simulink subsystem "SubSysWrappedState_Simplified7DOF"  (R2019b)
settings: Solver=VariableStepAuto  StartTime=0.0  StopTime=10.0  RelTol=1e-3
undefined symbols (not defined in the file): psi, psidot, X, xdot, Y, ydot
settings Model: Creator=yeyuan  LastModifiedBy=yeyuan

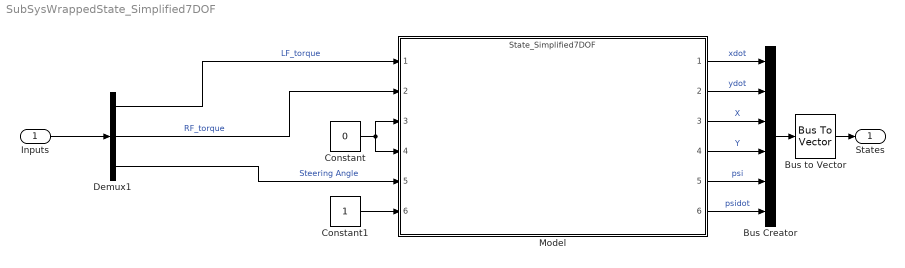
== system SubSysWrappedState_Simplified7DOF ==
  Inputs : Inport
  Bus Creator : BusCreator  Inputs=xdot,ydot,X,Y,psi,psidot
  Bus to Vector : BusToVector
  Constant : Constant  Value=0
  Constant1 : Constant
  Demux1 : Demux  Outputs=3
  Model : ModelReference  ModelNameDialog=State_Simplified7DOF.slx  SimulationMode=Normal  ModelReferenceVersion=1.13
  States : Outport  SignalName=States
  wires:
  Demux1/2 -> Model/2  "RF_torque"
  Model/5 -> Bus Creator/5  "psi"
  Model/6 -> Bus Creator/6  "psidot"
  Model/4 -> Bus Creator/4  "Y"
  Model/2 -> Bus Creator/2  "ydot"
  Demux1/3 -> Model/5  "Steering Angle"
  Constant1/1 -> Model/6
  Model/1 -> Bus Creator/1  "xdot"
  Constant/1 -> Model/4, Model/3
  Demux1/1 -> Model/1  "LF_torque"
  Model/3 -> Bus Creator/3  "X"
  Inputs/1 -> Demux1/1
  Bus Creator/1 -> Bus to Vector/1
  Bus to Vector/1 -> States/1
